simulink subsystem "Inputs_BatteryHV_Constant_refsub"  (R2026a)
settings: Solver=VariableStepAuto
undefined symbols (not defined in the file or in its folder): testParam, value
settings Model: Creator=isaacito  LastModifiedBy=isaacito
settings SimscapeCC: SimscapeNominalValues="[{\"value\":\"1\",\"unit\":\"A\"},{\"value\":\"1\",\"unit\":\"bar\"},{\"value\":\"1\",\"unit\":\"cm^2\"},{\"value\":\"1\",\"unit\":\"cm^3/s\"},{\"value\":\"1\",\"unit\":\"kJ/kg\"},{\"value\":\"1\",\"unit\":\"kW\"},{\"value\":\"1\",\"unit\":\"l\"},{\"value\":\"1\",\"unit\":\"N\"},{\"value\":\"1\",\"unit\":\"N*m\"},{\"value\":\"1\",\"unit\":\"V\"}]"  SimscapeLogType=none  SimscapeLogDataHistory=5000.0

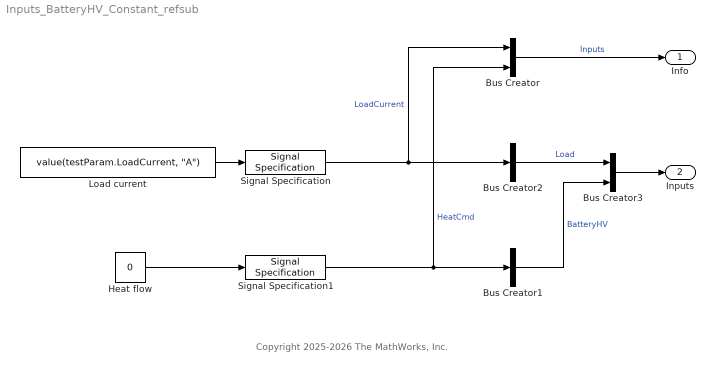
== system Inputs_BatteryHV_Constant_refsub ==
  note: Copyright 2025-2026 The MathWorks, Inc.
  Bus Creator : BusCreator  Inputs=2
  Bus Creator1 : BusCreator  Inputs=1
  Bus Creator2 : BusCreator  Inputs=1
  Bus Creator3 : BusCreator  Inputs=2
  Heat flow : Constant  Value=0
  Load current : Constant  Value="value(testParam.LoadCurrent, \"A\")"
  Signal Specification : SignalSpecification  Unit=A
  Signal Specification1 : SignalSpecification  Unit=W
  Info : Outport
  Inputs : Outport  Port=2
  wires:
  Bus Creator/1 -> Info/1  "Inputs"
  Load current/1 -> Signal Specification/1
  Bus Creator1/1 -> Bus Creator3/2  "BatteryHV"
  Bus Creator2/1 -> Bus Creator3/1  "Load"
  Bus Creator3/1 -> Inputs/1
  Heat flow/1 -> Signal Specification1/1
  Signal Specification/1 -> Bus Creator2/1, Bus Creator/1  "LoadCurrent"
  Signal Specification1/1 -> Bus Creator1/1, Bus Creator/2  "HeatCmd"
